simulink model "C_LQR"  (R2020b)
settings: Solver=VariableStepAuto  StartTime=0.0  StopTime=10  RelTol=1e-3
undefined symbols (not defined in the file): K1, K2, K3, K4, K5, sysE, sysM
settings Model: Creator=andre  LastModifiedBy=andre

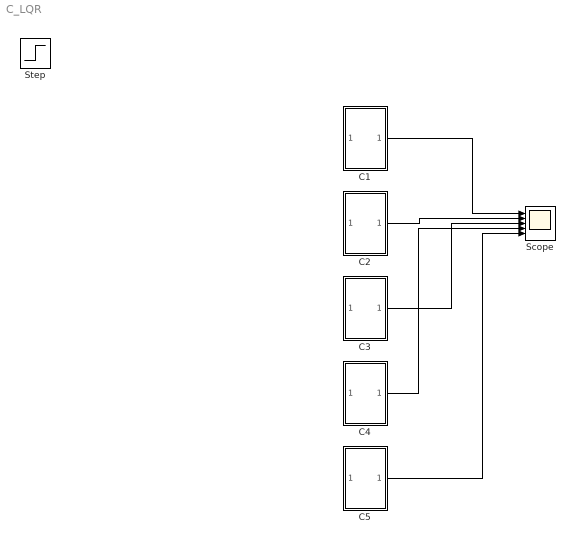
== system C_LQR ==
  C1 : Subsystem
  C2 : Subsystem
  C3 : Subsystem
  C4 : Subsystem
  C5 : Subsystem
  Scope : Scope  NumInputPorts=5
  Step : Step  Time=10  Before=1  After=0  SampleTime=0
  wires:
  C1/1(Out1) -> Scope/1
  C2/1(Out1) -> Scope/2
  C3/1(Out1) -> Scope/3
  C4/1(Out1) -> Scope/4
  C5/1(Out1) -> Scope/5

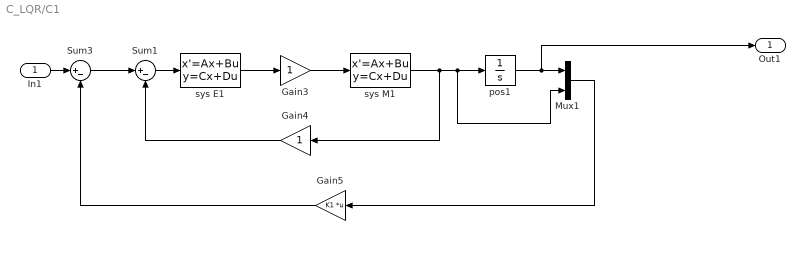
== system C_LQR/C1 ==
  In1 : Inport
  Gain3 : Gain
  Gain4 : Gain
  Gain5 : Gain  Gain=K1  Multiplication=Matrix(K*u)
  Mux1 : Mux  Inputs=2
  Sum1 : Sum  Inputs=|+-
  Sum3 : Sum  Inputs=|+-
  pos1 : Integrator  InitialCondition=1
  sys E1 : StateSpace  A=sysE.A  B=sysE.B  C=sysE.C  D=sysE.D  InitialCondition=0
  sys M1 : StateSpace  A=sysM.A  B=sysM.B  C=sysM.C  D=sysM.D  InitialCondition=0
  Out1 : Outport
  wires:
  sys E1/1 -> Gain3/1
  Sum1/1 -> sys E1/1
  pos1/1 -> Out1/1, Mux1/1
  Gain4/1 -> Sum1/2
  Gain3/1 -> sys M1/1
  sys M1/1 -> Mux1/2, pos1/1, Gain4/1
  Gain5/1 -> Sum3/2
  Sum3/1 -> Sum1/1
  Mux1/1 -> Gain5/1
  In1/1 -> Sum3/1

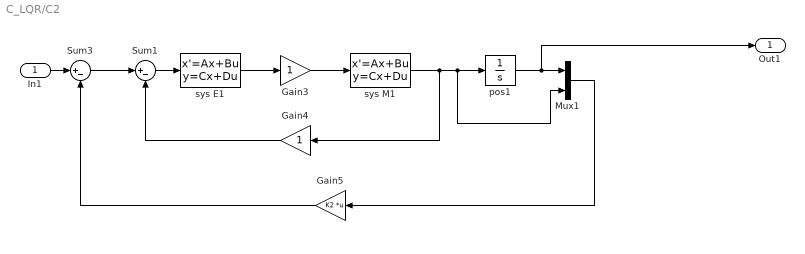
== system C_LQR/C2 ==
  In1 : Inport
  Gain3 : Gain
  Gain4 : Gain
  Gain5 : Gain  Gain=K2  Multiplication=Matrix(K*u)
  Mux1 : Mux  Inputs=2
  Sum1 : Sum  Inputs=|+-
  Sum3 : Sum  Inputs=|+-
  pos1 : Integrator  InitialCondition=1
  sys E1 : StateSpace  A=sysE.A  B=sysE.B  C=sysE.C  D=sysE.D  InitialCondition=0
  sys M1 : StateSpace  A=sysM.A  B=sysM.B  C=sysM.C  D=sysM.D  InitialCondition=0
  Out1 : Outport
  wires:
  sys E1/1 -> Gain3/1
  Sum1/1 -> sys E1/1
  pos1/1 -> Out1/1, Mux1/1
  Gain4/1 -> Sum1/2
  Gain3/1 -> sys M1/1
  sys M1/1 -> Mux1/2, pos1/1, Gain4/1
  Gain5/1 -> Sum3/2
  Sum3/1 -> Sum1/1
  Mux1/1 -> Gain5/1
  In1/1 -> Sum3/1

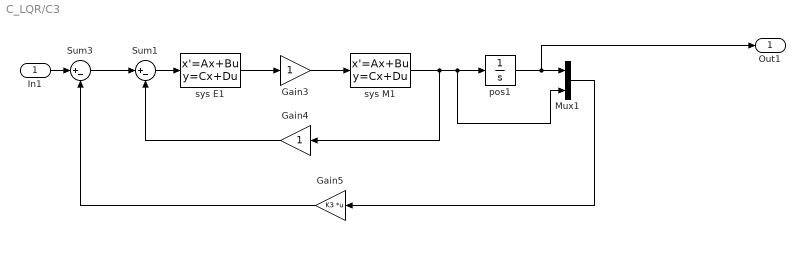
== system C_LQR/C3 ==
  In1 : Inport
  Gain3 : Gain
  Gain4 : Gain
  Gain5 : Gain  Gain=K3  Multiplication=Matrix(K*u)
  Mux1 : Mux  Inputs=2
  Sum1 : Sum  Inputs=|+-
  Sum3 : Sum  Inputs=|+-
  pos1 : Integrator  InitialCondition=1
  sys E1 : StateSpace  A=sysE.A  B=sysE.B  C=sysE.C  D=sysE.D  InitialCondition=0
  sys M1 : StateSpace  A=sysM.A  B=sysM.B  C=sysM.C  D=sysM.D  InitialCondition=0
  Out1 : Outport
  wires:
  sys E1/1 -> Gain3/1
  Sum1/1 -> sys E1/1
  pos1/1 -> Out1/1, Mux1/1
  Gain4/1 -> Sum1/2
  Gain3/1 -> sys M1/1
  sys M1/1 -> Mux1/2, pos1/1, Gain4/1
  Gain5/1 -> Sum3/2
  Sum3/1 -> Sum1/1
  Mux1/1 -> Gain5/1
  In1/1 -> Sum3/1

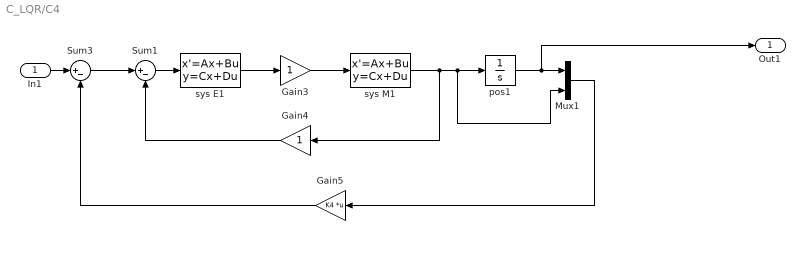
== system C_LQR/C4 ==
  In1 : Inport
  Gain3 : Gain
  Gain4 : Gain
  Gain5 : Gain  Gain=K4  Multiplication=Matrix(K*u)
  Mux1 : Mux  Inputs=2
  Sum1 : Sum  Inputs=|+-
  Sum3 : Sum  Inputs=|+-
  pos1 : Integrator  InitialCondition=1
  sys E1 : StateSpace  A=sysE.A  B=sysE.B  C=sysE.C  D=sysE.D  InitialCondition=0
  sys M1 : StateSpace  A=sysM.A  B=sysM.B  C=sysM.C  D=sysM.D  InitialCondition=0
  Out1 : Outport
  wires:
  sys E1/1 -> Gain3/1
  Sum1/1 -> sys E1/1
  pos1/1 -> Out1/1, Mux1/1
  Gain4/1 -> Sum1/2
  Gain3/1 -> sys M1/1
  sys M1/1 -> Mux1/2, pos1/1, Gain4/1
  Gain5/1 -> Sum3/2
  Sum3/1 -> Sum1/1
  Mux1/1 -> Gain5/1
  In1/1 -> Sum3/1

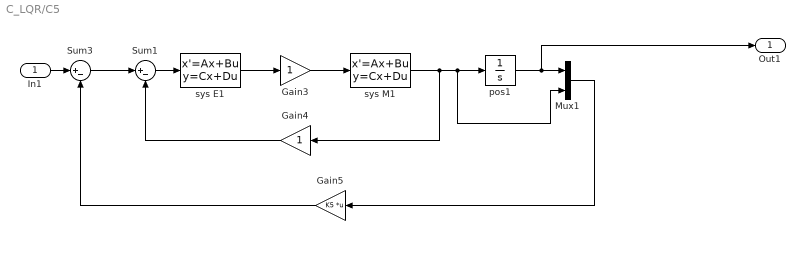
== system C_LQR/C5 ==
  In1 : Inport
  Gain3 : Gain
  Gain4 : Gain
  Gain5 : Gain  Gain=K5  Multiplication=Matrix(K*u)
  Mux1 : Mux  Inputs=2
  Sum1 : Sum  Inputs=|+-
  Sum3 : Sum  Inputs=|+-
  pos1 : Integrator  InitialCondition=1
  sys E1 : StateSpace  A=sysE.A  B=sysE.B  C=sysE.C  D=sysE.D  InitialCondition=0
  sys M1 : StateSpace  A=sysM.A  B=sysM.B  C=sysM.C  D=sysM.D  InitialCondition=0
  Out1 : Outport
  wires:
  sys E1/1 -> Gain3/1
  Sum1/1 -> sys E1/1
  pos1/1 -> Out1/1, Mux1/1
  Gain4/1 -> Sum1/2
  Gain3/1 -> sys M1/1
  sys M1/1 -> Mux1/2, pos1/1, Gain4/1
  Gain5/1 -> Sum3/2
  Sum3/1 -> Sum1/1
  Mux1/1 -> Gain5/1
  In1/1 -> Sum3/1
